simulink subsystem "Antenna"  (R2022b)
settings: Solver=VariableStepAuto  StartTime=0.0  StopTime=10.0  RelTol=1e-3
undefined symbols (not defined in the file): Azimuth_initial_angle, Elevation_initial_angle, J_azimuth, J_elevation
settings Model: Creator=Maxim Kozlov  LastModifiedBy=Maxim Kozlov
settings OptimizationCC: ReuseModelBlockBuffer=on

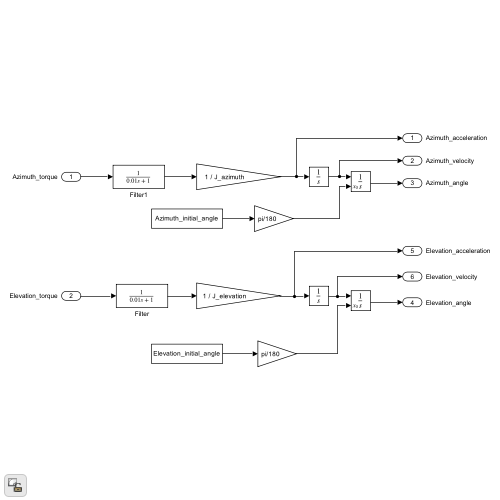
[thumbnail: Simulink's stored preview of the top-level diagram]
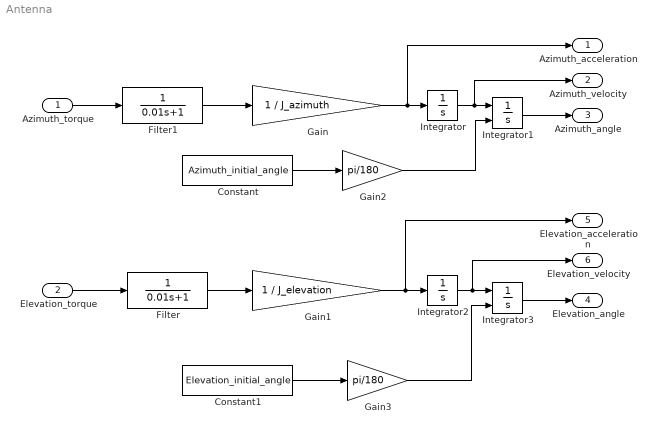
== system Antenna ==
  Azimuth_torque : Inport
  Elevation_torque : Inport  Port=2
  Constant : Constant  Value=Azimuth_initial_angle
  Constant1 : Constant  Value=Elevation_initial_angle
  Filter : TransferFcn  Denominator=[0.01 1]
  Filter1 : TransferFcn  Denominator=[0.01 1]
  Gain : Gain  Gain=1 / J_azimuth
  Gain1 : Gain  Gain=1 / J_elevation
  Gain2 : Gain  Gain=pi/180
  Gain3 : Gain  Gain=pi/180
  Integrator : Integrator
  Integrator1 : Integrator  InitialConditionSource=external
  Integrator2 : Integrator
  Integrator3 : Integrator  InitialConditionSource=external
  Azimuth_acceleration : Outport
  Azimuth_velocity : Outport  Port=2
  Azimuth_angle : Outport  Port=3
  Elevation_angle : Outport  Port=4
  Elevation_acceleration : Outport  Port=5
  Elevation_velocity : Outport  Port=6
  wires:
  Integrator2/1 -> Integrator3/1, Elevation_velocity/1
  Integrator1/1 -> Azimuth_angle/1
  Integrator/1 -> Integrator1/1, Azimuth_velocity/1
  Integrator3/1 -> Elevation_angle/1
  Azimuth_torque/1 -> Filter1/1
  Elevation_torque/1 -> Filter/1
  Constant/1 -> Gain2/1
  Constant1/1 -> Gain3/1
  Gain2/1 -> Integrator1/2
  Gain3/1 -> Integrator3/2
  Gain1/1 -> Integrator2/1, Elevation_acceleration/1
  Gain/1 -> Integrator/1, Azimuth_acceleration/1
  Filter1/1 -> Gain/1
  Filter/1 -> Gain1/1
